simulink model "prviModel"  (R2020a)
settings: Solver=VariableStepAuto  StartTime=0.0  StopTime=10.0  RelTol=1e-3
settings Model: Creator=Vedran  LastModifiedBy=Vedran

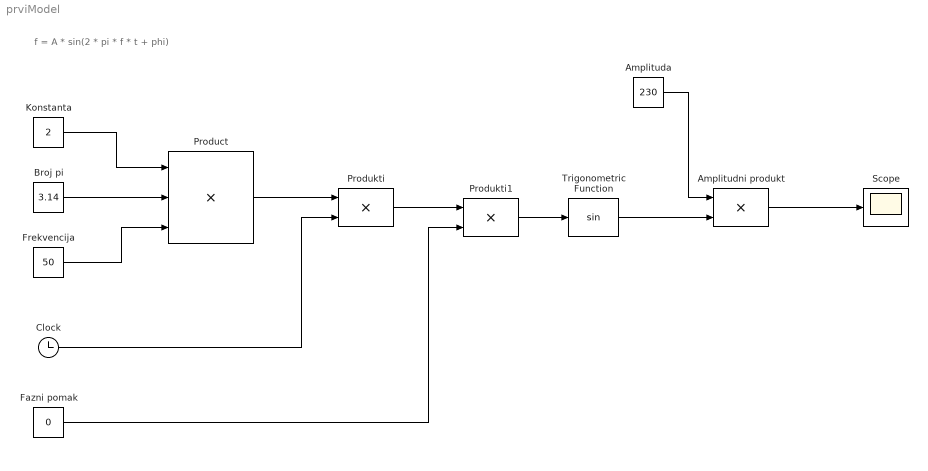
== system prviModel ==
  note: f = A * sin(2 * pi * f * t + phi)
  Amplituda : Constant  Value=230
  Amplitudni produkt : Product
  Broj pi : Constant  Value=3.14
  Clock : Clock
  Fazni pomak : Constant  Value=0
  Frekvencija : Constant  Value=50
  Konstanta : Constant  Value=2
  Product : Product  Inputs=3
  Produkti : Product
  Produkti1 : Product
  Scope : Scope
  Trigonometric Function : Trigonometry
  wires:
  Konstanta/1 -> Product/1
  Broj pi/1 -> Product/2
  Frekvencija/1 -> Product/3
  Product/1 -> Produkti/1
  Clock/1 -> Produkti/2
  Fazni pomak/1 -> Produkti1/2
  Produkti/1 -> Produkti1/1
  Produkti1/1 -> Trigonometric Function/1
  Trigonometric Function/1 -> Amplitudni produkt/2
  Amplituda/1 -> Amplitudni produkt/1
  Amplitudni produkt/1 -> Scope/1
